simulink model "systemnnpredictive"  (R2021a)
settings: Solver=VariableStepAuto  StartTime=0.0  StopTime=10  FixedStep=0.01  RelTol=1e-3
undefined symbols (not defined in the file or in its folder): daq
libraries: daqlib x2, neural x1
settings Model: Creator=ASUS  LastModifiedBy=USER

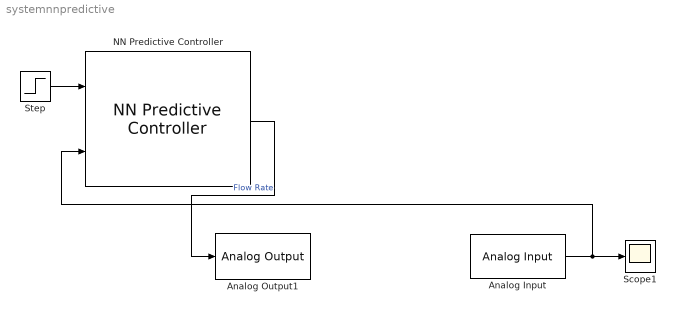
== system systemnnpredictive ==
  Analog Input : daqlib/Analog Input  DeviceMenu=(none)  Device=ni Dev3 (USB-6221)  ObjConstructor=daq.createSession('ni')  NChannelsSelected=16  Channels=1$ai0$$Dev3$1$4$3$1$#1$ai1$$Dev3$1$4$3$1$#1$ai2$$Dev3$1$4$3$1$#1$ai3$$Dev3$1$4$3$1$#1$ai4$$Dev3$1$4$3$1$#1$ai5$$Dev3$1$4$3$1$#1$ai6$$Dev3$1$4$3$1$#1$ai7$$Dev3$1$4$3$1$#1$ai8$$Dev3$1$4$1$1$#1$ai9$$Dev3$1$4$1$1$#1$ai10$$Dev3$1$4$1$1$#1$ai11$$Dev3$1$4$1$1$#1$ai12$$Dev3$1$4$1$1$#1$ai13$$Dev3$1$4$1$1$#1$ai14$$Dev3$1$4$1$1$#1$ai15$$Dev3$1$4$1$1$#  NPorts=1 for all channels  SampleRate=1000  ActualRate=1000  ScansPerTrigger=50  OutputTimestamp=off  AcqMode=0  NumFrameBuffer=100  OutputTriggertime=off
      settings: SourceProductBaseCode=DA
  Analog Output1 : daqlib/Analog Output  DeviceMenu=(none)  Device=ni Dev3 (USB-6221)  ObjConstructor=daq.createSession('ni')  NChannelsSelected=2  Channels=1$ao0$$Dev3$1$1$N/A$#1$ao1$$Dev3$1$1$N/A$#  NPorts=1 for all channels  SampleRate=1000  ActualRate=1000
      settings: SourceProductBaseCode=DA
  NN Predictive Controller : neural/Control Systems/NN Predictive Controller  epochs=200  minp=-9.8435941286133026296  maxp=9.9231222259373872419  mint=-4605.5325534448220424  maxt=9.9231222259373872419  Normalize=0  IW=[57.977779220742711175 33.445696709063632568;125.46566152952536299 114.6993096470896063;96.609483205571734743 -44.584873053539766374;35.144855900631213785 -25.356417340148603046;-33.864199342534874404 47.069237173016801989;2865.1577828774252339 2637.9122090658429443;81.109078112036044672 -10.464446633552194399;255.73329793887373285 -7.403730076895680412;88.766144213046999312 56.85784285299158114;-314.90438914323118524 -28.519573350562499314]  LW1_2=[108.51391976768117331 -109.80343773919329919;276.20153574321943779 -281.46841030244468129;-315.14715477380883613 -206.13939166202720799;-459.19700205843787444 -420.40966564235787928;-155.20645622924558893 -510.37349569966647778;-513.12429174221745143 504.83916552523743349;-11.548204281666505366 7.6204621838846122728;-50.682287894702170661 36.51843862672370733;4.7388794330520944698 -5.406183242201844763;-118.80481171290681175 115.0131616898893725]  LW2_1=[2.7099382327127514714 -370.18310995725761359 -205.80319637630404372 -644.44197501492112679 -606.92766654297020068 -381.34810485303336236 -542.25652152369661962 -843.37749638651894202 -311.89328360075427327 -835.10778215240668487]  B1=[30.468316242156586071;-20.737061146359636155;74.949241484402548963;-26.0610466596042194;211.98235493420600051;1211.2835070018859369;6.2359923189019665912;147.55670930293865695;103.37495869043871721;-15.882788785289717381]  B2=1440.0993441398713912  max_i_int=1  min_i_int=0.5  limit_output=0  max_output=Inf  min_output=-Inf  Use_Previous_Weights=1  N2=30  Nu=2  Ts=0.2  rho=0.05  alpha=0.001  csrchfun=csrchbac  maxiter=2  S1=10  Ni=2  Nj=2  sim_file=cstr  trainfun=trainlm  Use_validation=1  Use_Testing=1  max_i=10  min_i=-10  sam_training=1000
      settings: SourceProductBaseCode=NN
  Scope1 : Scope
  Step : Step  Time=0  After=11  SampleTime=0
  wires:
  Step/1 -> NN Predictive Controller/1
  Analog Input/1 -> NN Predictive Controller/2, Scope1/1
  NN Predictive Controller/1 -> Analog Output1/1  "Flow Rate"
